simulink model "MainPlanevsRainCameras"  (R2020a)
settings: Solver=FixedStepDiscrete  StartTime=0.0  StopTime=20  RelTol=1e-3
model workspace (MAT data in the model file):
  firstWarning = 0
  originalScenarioChecksum = '4AECC2AEC181DD8EA774641D9E64C004'
undefined symbols (not defined in the file): driving
libraries: drivingscenarioandsensors x28
(part 1 of 6)
settings Model: Creator=Monster  LastModifiedBy=Monster

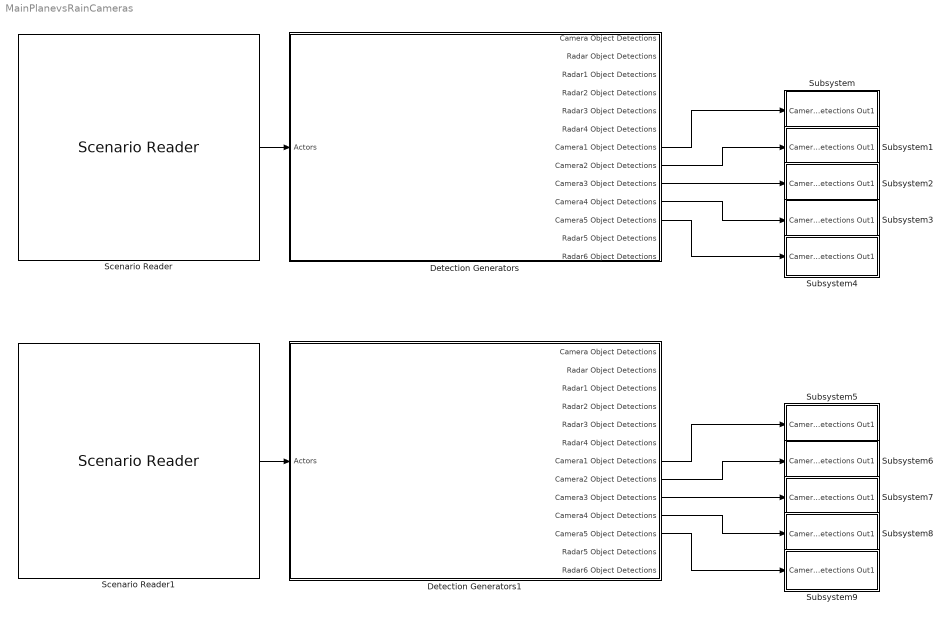
== system MainPlanevsRainCameras ==
  Detection Generators : Subsystem
  Detection Generators1 : Subsystem
  Scenario Reader : drivingscenarioandsensors/Scenario Reader  ScenarioSource=From file  ScenarioFileName=C:\Users\Monster\Desktop\Oytun Ozan\Ee 402\Main Track Rain.mat  ScenarioVariableName=scenario  OutputCoordinateSystem=Vehicle coordinates  EgoVehicleSource=Scenario  OrientVehiclesOnRoad=off  EgoVehicleActorID=1  OutputEgoVehiclePose=off  SampleTime=0.1  LaneBoundaryOutput=None  LaneBoundaryDistance=0:0.5:9.5  LaneBoundaryLocation=Center of lane markings  BusNameSource=Auto  BusName=BusActors  BusName2Source=Auto  BusName2=BusLaneBoundaries  BusName3Source=Auto  BusName3=BusEgoActor  ShowCoordinateLabels=on  SimulateUsing=Interpreted execution
  Scenario Reader1 : drivingscenarioandsensors/Scenario Reader  ScenarioSource=From file  ScenarioFileName=C:\Users\Monster\Desktop\Oytun Ozan\Ee 402\Main Track.mat  ScenarioVariableName=scenario  OutputCoordinateSystem=Vehicle coordinates  EgoVehicleSource=Scenario  OrientVehiclesOnRoad=off  EgoVehicleActorID=1  OutputEgoVehiclePose=off  SampleTime=0.1  LaneBoundaryOutput=None  LaneBoundaryDistance=0:0.5:9.5  LaneBoundaryLocation=Center of lane markings  BusNameSource=Auto  BusName=BusActors  BusName2Source=Auto  BusName2=BusLaneBoundaries  BusName3Source=Auto  BusName3=BusEgoActor  ShowCoordinateLabels=on  SimulateUsing=Interpreted execution
  Subsystem : Subsystem
  Subsystem1 : Subsystem
  Subsystem2 : Subsystem
  Subsystem3 : Subsystem
  Subsystem4 : Subsystem
  Subsystem5 : Subsystem
  Subsystem6 : Subsystem
  Subsystem7 : Subsystem
  Subsystem8 : Subsystem
  Subsystem9 : Subsystem
  wires:
  Scenario Reader/1 -> Detection Generators/1(Actors)
  Detection Generators/9(Camera3 Object Detections) -> Subsystem2/1(Camera3 Object Detections)
  Detection Generators/8(Camera2 Object Detections) -> Subsystem1/1(Camera2 Object Detections)
  Detection Generators/7(Camera1 Object Detections) -> Subsystem/1(Camera1 Object Detections)
  Detection Generators/10(Camera4 Object Detections) -> Subsystem3/1(Camera4 Object Detections)
  Detection Generators/11(Camera5 Object Detections) -> Subsystem4/1(Camera5 Object Detections)
  Scenario Reader1/1 -> Detection Generators1/1(Actors)
  Detection Generators1/9(Camera3 Object Detections) -> Subsystem7/1(Camera3 Object Detections)
  Detection Generators1/8(Camera2 Object Detections) -> Subsystem6/1(Camera2 Object Detections)
  Detection Generators1/10(Camera4 Object Detections) -> Subsystem8/1(Camera4 Object Detections)
  Detection Generators1/11(Camera5 Object Detections) -> Subsystem9/1(Camera5 Object Detections)
  Detection Generators1/7(Camera1 Object Detections) -> Subsystem5/1(Camera1 Object Detections)
